simulink model "powellsMethodMin_th"  (R2018b)
settings: Solver=ode8  StartTime=0.0  StopTime=0  FixedStep=0.5  RelTol=1e-3  EnableMultiTasking=on
values from neighbouring files (symbols this model uses):
  rCentroidBotA = tsc.rCentroidBotA.Data(:,:,timeIndex)    [snellsMin_ts.m]
  rCentroidBotB = tsc.rCentroidBotB.Data(:,:,timeIndex)    [snellsMin_ts.m]
  rCentroidSide = tsc.rCentroidSide.Data(:,:,timeIndex)    [snellsMin_ts.m]
  rCentroidSlant = tsc.rCentroidSlant.Data(:,:,timeIndex)    [snellsMin_ts.m]
  uCentroidBotA = tsc.uCentroidBotA.Data(:,:,timeIndex)    [snellsMin_ts.m]
  uCentroidBotB = tsc.uCentroidBotB.Data(:,:,timeIndex)    [snellsMin_ts.m]
  uCentroidSide = tsc.uCentroidSide.Data(:,:,timeIndex)    [snellsMin_ts.m]
  uCentroidSlant = tsc.uCentroidSlant.Data(:,:,timeIndex)    [snellsMin_ts.m]
libraries: powellsMethodMin_ul x1
settings Model: Creator=MAE-NCSUCORE  LastModifiedBy=MAE-NCSUCORE
settings SolverCC: ConcurrentTasks=on  AutoInsertRateTranBlk=on
settings DataIOCC: SaveFormat=StructureWithTime
settings OptimizationCC: BlockReduction=off  OptimizeBlockIOStorage=off  BufferReuse=off  GlobalBufferReuse=off  ExpressionFolding=off  LocalBlockOutputs=off  OptimizeDataStoreBuffers=off  BusAssignmentInplaceUpdate=off
settings HardwareCC: ProdBitPerPointer=32  ProdBitPerSizeT=32  ProdBitPerPtrDiffT=32  ProdLargestAtomicFloat=None  ProdWordSize=32  ProdLongLongMode=on  ProdHWDeviceType=Generic->32-bit x86 compatible
settings RTWCC: Description=Generic Real-Time Target  RTWCompilerOptimization=on
settings GRTTargetCC: TargetLangStandard=C89/C90 (ANSI)

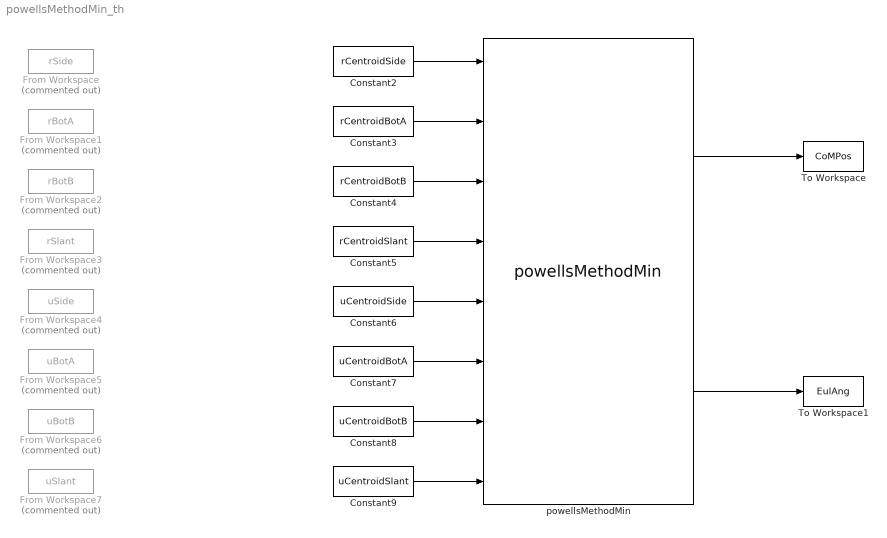
== system powellsMethodMin_th ==
  Constant2 : Constant  Value=rCentroidSide
  Constant3 : Constant  Value=rCentroidBotA
  Constant4 : Constant  Value=rCentroidBotB
  Constant5 : Constant  Value=rCentroidSlant
  Constant6 : Constant  Value=uCentroidSide
  Constant7 : Constant  Value=uCentroidBotA
  Constant8 : Constant  Value=uCentroidBotB
  Constant9 : Constant  Value=uCentroidSlant
  From Workspace : FromWorkspace  Commented=on  VariableName=rSide  SampleTime=0
  From Workspace1 : FromWorkspace  Commented=on  VariableName=rBotA  SampleTime=0
  From Workspace2 : FromWorkspace  Commented=on  VariableName=rBotB  SampleTime=0
  From Workspace3 : FromWorkspace  Commented=on  VariableName=rSlant  SampleTime=0
  From Workspace4 : FromWorkspace  Commented=on  VariableName=uSide  SampleTime=0
  From Workspace5 : FromWorkspace  Commented=on  VariableName=uBotA  SampleTime=0
  From Workspace6 : FromWorkspace  Commented=on  VariableName=uBotB  SampleTime=0
  From Workspace7 : FromWorkspace  Commented=on  VariableName=uSlant  SampleTime=0
  To Workspace : ToWorkspace  VariableName=CoMPos  SaveFormat=Timeseries  SampleTime=-1
  To Workspace1 : ToWorkspace  VariableName=EulAng  SaveFormat=Timeseries  SampleTime=-1
  powellsMethodMin : powellsMethodMin_ul/powellsMethodMin  sideDotPosVec_cm=params.sideDotPosVec_cm.Value'  botADotPosVec_cm=params.botADotPosVec_cm.Value'  botBDotPosVec_cm=params.botBDotPosVec_cm.Value'  initialCoMPositionVec_cm=initialCoMPositionVec_cm  initialEulerAngles_rad=initialEulerAngles_rad
  wires:
  powellsMethodMin/1 -> To Workspace/1
  powellsMethodMin/2 -> To Workspace1/1
  Constant2/1 -> powellsMethodMin/1
  Constant3/1 -> powellsMethodMin/2
  Constant4/1 -> powellsMethodMin/3
  Constant5/1 -> powellsMethodMin/4
  Constant6/1 -> powellsMethodMin/5
  Constant7/1 -> powellsMethodMin/6
  Constant8/1 -> powellsMethodMin/7
  Constant9/1 -> powellsMethodMin/8
